simulink model "Joystick"  (R2016b)
settings: Solver=VariableStepAuto  StartTime=0.0  StopTime=30  RelTol=1e-3
values from neighbouring files (symbols this model uses):
  a = -real(s1) + imag(s1)/tan(angle(s1+b) - theta)    [RLDesignJoystick.m]
  a1 = b1/K    [RLDesignJoystick.m]
  b = 1.2*bb/I    (= 0.4)    [RLDesignJoystick.m]
  b1 = -real(s1)/150    [RLDesignJoystick.m]
  bb = 0.254    [RLDesignJoystick.m]
  I = 0.762    [RLDesignJoystick.m]
  K0 = abs(s1+a)/abs(Gs1)/abs(s1+b)    [RLDesignJoystick.m]
  K1 = 1/abs(Gs1)    [RLDesignJoystick.m]
settings Model: Creator=KvonEllenrieder  LastModifiedBy=KvonEllenrieder

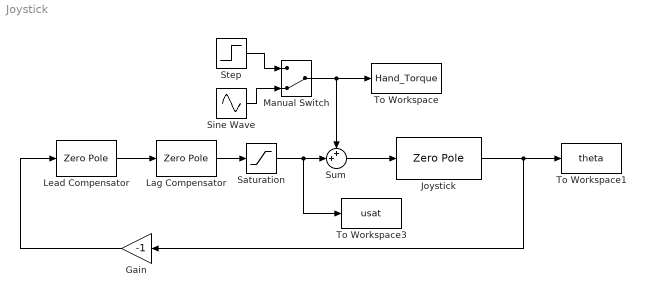
== system Joystick ==
  Gain : Gain  Gain=-1
  Joystick : ZeroPole  Zeros=[]  Poles=[0, -bb/I]  Gain=I
  Lag Compensator : ZeroPole  Zeros=[-b1]  Poles=[-a1]  Gain=[K1]
  Lead Compensator : ZeroPole  Zeros=[-b]  Poles=[-a]  Gain=[K0]
  Manual Switch : ManualSwitch  CurrentSetting=0
  Saturation : Saturate  UpperLimit=3  LowerLimit=-3
  Sine Wave : Sin  SampleTime=0
  Step : Step  Time=3  SampleTime=0
  Sum : Sum  Inputs=++|
  To Workspace : ToWorkspace  VariableName=Hand_Torque  SaveFormat=Timeseries  SampleTime=-1
  To Workspace1 : ToWorkspace  VariableName=theta  SaveFormat=Timeseries  SampleTime=-1
  To Workspace3 : ToWorkspace  VariableName=usat  SaveFormat=Timeseries  SampleTime=-1
  wires:
  Manual Switch/1 -> To Workspace/1, Sum/1
  Joystick/1 -> Gain/1, To Workspace1/1
  Lead Compensator/1 -> Lag Compensator/1
  Sum/1 -> Joystick/1
  Gain/1 -> Lead Compensator/1
  Saturation/1 -> To Workspace3/1, Sum/2
  Lag Compensator/1 -> Saturation/1
  Step/1 -> Manual Switch/1
  Sine Wave/1 -> Manual Switch/2
